simulink model "ADHW2p2"  (R2022a)
settings: Solver=VariableStepAuto  StartTime=0.0  StopTime=100.0  RelTol=1e-3
settings Model: Creator=izacu  LastModifiedBy=izacu

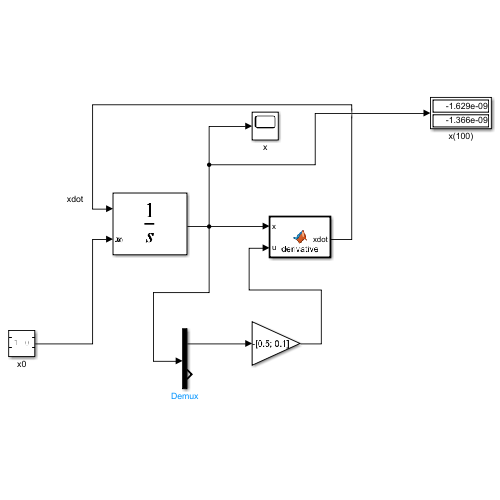
[thumbnail: Simulink's stored preview of the top-level diagram]
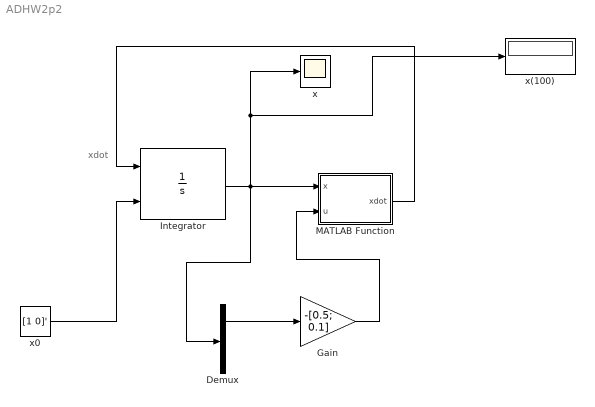
== system ADHW2p2 ==
  note: xdot
  Demux : Demux  Outputs=2
  Gain : Gain  Gain=-[0.5; 0.1]
  Integrator : Integrator  InitialConditionSource=external
  MATLAB Function : MATLAB Function  TreatAsAtomicUnit=on
  x : Scope
  x(100) : Display
  x0 : Constant  Value=[1 0]'
  wires:
  x0/1 -> Integrator/2
  Integrator/1 -> x(100)/1, x/1, Demux/1, MATLAB Function/1(x)
  Demux/1 -> Gain/1
  Gain/1 -> MATLAB Function/2(u)
  MATLAB Function/1(xdot) -> Integrator/1

== matlab function ADHW2p2/MATLAB Function ==
  data: x input; u input; xdot output
function xdot = derivative(x,u)
A = [0 1; -1 0.1];
xdot = A*x + u;
